simulink library "halin"  (R2021b)
settings: Solver=VariableStepAuto  StartTime=0.0  StopTime=10.0  RelTol=1e-3
undefined symbols (not defined in the file): KHAL_CAN1ABM1E2E_flg, KHAL_CAN1ESC1E2E_flg, KHAL_CAN1ESC5E2E_flg, KHAL_CAN1ESC7E2E_flg, KHAL_CAN1FCM2E2E_flg, KHAL_CAN1FCM3E2E_flg, KHAL_CAN1FCM4E2E_flg, KHAL_CAN3BMS1E2E_flg, KHAL_CAN3BMS6E2E_flg, KHAL_CAN3CCU1E2E_flg, KHAL_CAN3CCU2E2E_flg, KHAL_CAN3MCUF1E2E_flg, KHAL_CAN3MCUR1E2E_flg, KHAL_CAN3Shifter1E2E_flg, TRUE
libraries: simulink x420, FVT_lib x149, hcu_lib x49
(part 7 of 14)

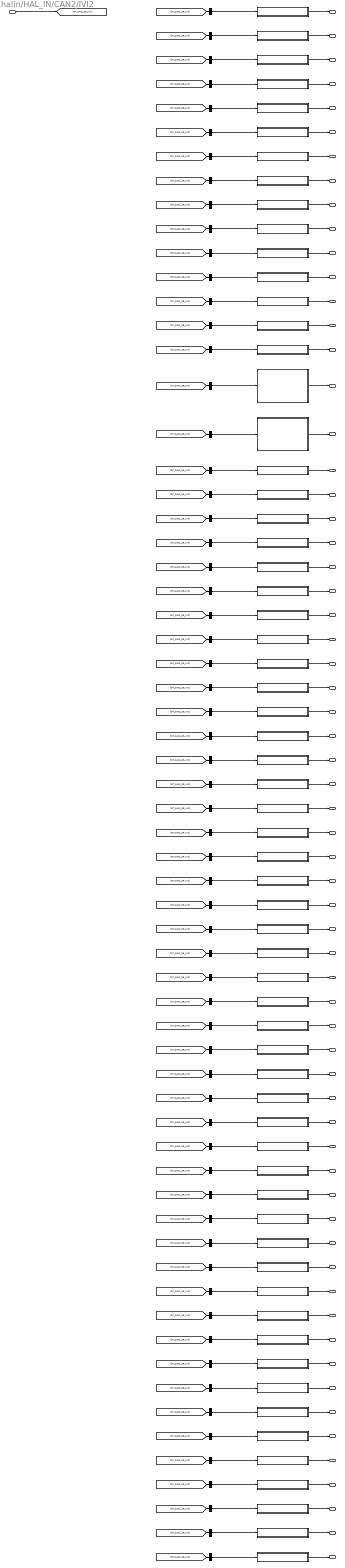
== system halin/HAL_IN/CAN2/IVI2 ==
  DT_CAN2_SG_IVI2 : Inport
  AVMErrSTA : Subsystem
  AVMOFFRecButt : Subsystem
  AVMParkingmode : Subsystem
  AVMparkingcancel : Subsystem
  AVMparkingexcute : Subsystem
  ApproachUnlockSW : Subsystem
  CAASSw : Subsystem
  CDLLockButt : Subsystem
  CDLUnlockButt : Subsystem
  DSEATantiset : Subsystem
  DSEATentryfunset : Subsystem
  DSEATventreq : Subsystem
  ESCSWCmd : Subsystem
  FSOffSw : Subsystem
  FollowMeSW : Subsystem
  GPSLAT : Subsystem
  GPSLONG : Subsystem
  HeadLampSW : Subsystem
  HoodLatchSW : Subsystem
  IVICreepSWReq : Subsystem
  IVIISAOffsetSpd : Subsystem
  IVINightModeSta : Subsystem
  IVIPTGModeSW : Subsystem
  IVIPTGOpenHeight : Subsystem
  IVIPTGStaSW : Subsystem
  IVIPTGUSStaSW : Subsystem
  IVIPWModeReq : Subsystem
  IVIPwrLockSW : Subsystem
  IVIPwroffreq : Subsystem
  IVIRRDefReq : Subsystem
  IVIReqV2L : Subsystem
  IVIScreen : Subsystem
  IVIStatus : Subsystem
  IVITriggerreq : Subsystem
  IVIWIMAINSW : Subsystem
  LDrvControlCommand : Subsystem
  LPasControlCommand : Subsystem
  LRLDControlCommand : Subsystem
  LRRDControlCommand : Subsystem
  MFRDNBrightReq : Subsystem
  OFFACMODE : Subsystem
  PSEATventreq : Subsystem
  PerdV2L : Subsystem
  RFogLampSW : Subsystem
  RollModeSWCmd : Subsystem
  RoomLampMode : Subsystem
  SOCV2LLimit : Subsystem
  SchedChgbutt : Subsystem
  SchedChgwake : Subsystem
  SenstivityPosition : Subsystem
  SetUnlockSingle : Subsystem
  TCSSWCmd : Subsystem
  TPMSCaliButt : Subsystem
  TPMSResButt : Subsystem
  TurnSwTimeSet : Subsystem
  WalkawayLockSW : Subsystem
  bus_selector : BusSelector  OutputSignals=CAN2_AVM_Err_STA
  bus_selector1 : BusSelector  OutputSignals=CAN2_AVM_OFF_Rec_Butt
  bus_selector10 : BusSelector  OutputSignals=CAN2_DSEAT_entryfun_set
  bus_selector11 : BusSelector  OutputSignals=CAN2_DSEAT_vent_req
  bus_selector12 : BusSelector  OutputSignals=CAN2_ESC_SW_Cmd
  bus_selector13 : BusSelector  OutputSignals=CAN2_FS_Off_Sw
  bus_selector14 : BusSelector  OutputSignals=CAN2_FollowMeSW
  bus_selector15 : BusSelector  OutputSignals=CAN2_GPS_LAT
  bus_selector16 : BusSelector  OutputSignals=CAN2_GPS_LONG
  bus_selector17 : BusSelector  OutputSignals=CAN2_HeadLampSW
  bus_selector18 : BusSelector  OutputSignals=CAN2_Hood_Latch_SW
  bus_selector19 : BusSelector  OutputSignals=CAN2_IVI_CreepSW_Req
  bus_selector2 : BusSelector  OutputSignals=CAN2_AVM_Parking_mode
  bus_selector20 : BusSelector  OutputSignals=CAN2_IVI_ISA_OffsetSpd
  bus_selector21 : BusSelector  OutputSignals=CAN2_IVI_Night_Mode_Sta
  bus_selector22 : BusSelector  OutputSignals=CAN2_IVI_PTG_Mode_SW
  bus_selector23 : BusSelector  OutputSignals=CAN2_IVI_PTG_Open_Height
  bus_selector24 : BusSelector  OutputSignals=CAN2_IVI_PTG_Sta_SW
  bus_selector25 : BusSelector  OutputSignals=CAN2_IVI_PTG_USSta_SW
  bus_selector26 : BusSelector  OutputSignals=CAN2_IVI_PW_Mode_Req
  bus_selector27 : BusSelector  OutputSignals=CAN2_IVI_PwrLockSW
  bus_selector28 : BusSelector  OutputSignals=CAN2_IVI_Pwroff_req
  bus_selector29 : BusSelector  OutputSignals=CAN2_IVI_RR_Def_Req
  bus_selector3 : BusSelector  OutputSignals=CAN2_AVM_parking_cancel
  bus_selector30 : BusSelector  OutputSignals=CAN2_IVI_Req_V2L
  bus_selector31 : BusSelector  OutputSignals=CAN2_IVI_Screen
  bus_selector32 : BusSelector  OutputSignals=CAN2_IVI_Status
  bus_selector33 : BusSelector  OutputSignals=CAN2_IVI_Trigger_req
  bus_selector34 : BusSelector  OutputSignals=CAN2_IVI_WI_MAIN_SW
  bus_selector35 : BusSelector  OutputSignals=CAN2_L_Drv_ControlCommand
  bus_selector36 : BusSelector  OutputSignals=CAN2_L_Pas_ControlCommand
  bus_selector37 : BusSelector  OutputSignals=CAN2_L_RLD_ControlCommand
  bus_selector38 : BusSelector  OutputSignals=CAN2_L_RRD_ControlCommand
  bus_selector39 : BusSelector  OutputSignals=CAN2_MFRD_N_Bright_Req
  bus_selector4 : BusSelector  OutputSignals=CAN2_AVM_parking_excute
  bus_selector40 : BusSelector  OutputSignals=CAN2_OFF_AC_MODE
  bus_selector41 : BusSelector  OutputSignals=CAN2_PSEAT_vent_req
  bus_selector42 : BusSelector  OutputSignals=CAN2_Perd_V2L
  bus_selector43 : BusSelector  OutputSignals=CAN2_RFogLampSW
  bus_selector44 : BusSelector  OutputSignals=CAN2_Roll_Mode_SW_Cmd
  bus_selector45 : BusSelector  OutputSignals=CAN2_RoomLampMode
  bus_selector46 : BusSelector  OutputSignals=CAN2_SOC_V2LLimit
  bus_selector47 : BusSelector  OutputSignals=CAN2_Sched_Chg_butt
  bus_selector48 : BusSelector  OutputSignals=CAN2_Sched_Chg_wake
  bus_selector49 : BusSelector  OutputSignals=CAN2_SenstivityPosition
  bus_selector5 : BusSelector  OutputSignals=CAN2_Approach_Unlock_SW
  bus_selector50 : BusSelector  OutputSignals=CAN2_SetUnlockSingle
  bus_selector51 : BusSelector  OutputSignals=CAN2_TCS_SW_Cmd
  bus_selector52 : BusSelector  OutputSignals=CAN2_TPMS_Cali_Butt
  bus_selector53 : BusSelector  OutputSignals=CAN2_TPMS_Res_Butt
  bus_selector54 : BusSelector  OutputSignals=CAN2_TurnSwTimeSet
  bus_selector55 : BusSelector  OutputSignals=CAN2_Walkaway_Lock_SW
  bus_selector56 : BusSelector  OutputSignals=CAN2_sigAirIntenZon1Req
  bus_selector57 : BusSelector  OutputSignals=CAN2_sigDfrstReq
  bus_selector58 : BusSelector  OutputSignals=CAN2_sigFaceReq
  bus_selector59 : BusSelector  OutputSignals=CAN2_sigFootReq
  bus_selector6 : BusSelector  OutputSignals=CAN2_CAAS_Sw
  bus_selector60 : BusSelector  OutputSignals=CAN2_sigRecircReq
  bus_selector61 : BusSelector  OutputSignals=CAN2_sigSetTempZon1Req
  bus_selector62 : BusSelector  OutputSignals=CAN2_sigSetTempZon2Req
  bus_selector7 : BusSelector  OutputSignals=CAN2_CDL_Lock_Butt
  bus_selector8 : BusSelector  OutputSignals=CAN2_CDL_Unlock_Butt
  bus_selector9 : BusSelector  OutputSignals=CAN2_DSEAT_anti_set
  sigAirIntenZon1Req : Subsystem
  sigDfrstReq : Subsystem
  sigFaceReq : Subsystem
  sigFootReq : Subsystem
  sigRecircReq : Subsystem
  sigSetTempZon1Req : Subsystem
  sigSetTempZon2Req : Subsystem
  VHAL_AVMErrSTA_flg : Outport
  VHAL_AVMOFFRecButt_flg : Outport  Port=2
  VHAL_AVMParkingmode_enum : Outport  Port=3
  VHAL_AVMparkingcancel_enum : Outport  Port=4
  VHAL_AVMparkingexcute_enum : Outport  Port=5
  VHAL_ApproachUnlockSW_flg : Outport  Port=6
  VHAL_CAASSw_enum : Outport  Port=7
  VHAL_CDLLockButt_flg : Outport  Port=8
  VHAL_CDLUnlockButt_flg : Outport  Port=9
  VHAL_DSEATantiset_flg : Outport  Port=10
  VHAL_DSEATentryfunset_flg : Outport  Port=11
  VHAL_DSEATventreq_enum : Outport  Port=12
  VHAL_ESCSWCmd_enum : Outport  Port=13
  VHAL_FSOffSw_enum : Outport  Port=14
  VHAL_FollowMeSW_flg : Outport  Port=15
  VHAL_GPSLAT_s : Outport  Port=16
  VHAL_GPSLONG_enum : Outport  Port=17
  VHAL_HeadLampSW_enum : Outport  Port=18
  VHAL_HoodLatchSW_enum : Outport  Port=19
  VHAL_IVICreepSWReq_flg : Outport  Port=20
  VHAL_IVIISAOffsetSpd_enum : Outport  Port=21
  VHAL_IVINightModeSta_flg : Outport  Port=22
  VHAL_IVIPTGModeSW_enum : Outport  Port=23
  VHAL_IVIPTGOpenHeight_enum : Outport  Port=24
  VHAL_IVIPTGStaSW_enum : Outport  Port=25
  VHAL_IVIPTGUSStaSW_flg : Outport  Port=26
  VHAL_IVIPWModeReq_enum : Outport  Port=27
  VHAL_IVIPwrLockSW_enum : Outport  Port=28
  VHAL_IVIPwroffreq_flg : Outport  Port=29
  VHAL_IVIRRDefReq_flg : Outport  Port=30
  VHAL_IVIReqV2L_flg : Outport  Port=31
  VHAL_IVIScreen_enum : Outport  Port=32
  VHAL_IVIStatus_flg : Outport  Port=33
  VHAL_IVITriggerreq_flg : Outport  Port=34
  VHAL_IVIWIMAINSW_flg : Outport  Port=35
  VHAL_LDrvControlCommand_pct : Outport  Port=36
  VHAL_LPasControlCommand_pct : Outport  Port=37
  VHAL_LRLDControlCommand_pct : Outport  Port=38
  VHAL_LRRDControlCommand_pct : Outport  Port=39
  VHAL_MFRDNBrightReq_pct : Outport  Port=40
  VHAL_OFFACMODE_enum : Outport  Port=41
  VHAL_PSEATventreq_enum : Outport  Port=42
  VHAL_PerdV2L_enum : Outport  Port=43
  VHAL_RFogLampSW_flg : Outport  Port=44
  VHAL_RollModeSWCmd_enum : Outport  Port=45
  VHAL_RoomLampMode_flg : Outport  Port=46
  VHAL_SOCV2LLimit_pct : Outport  Port=47
  VHAL_SchedChgbutt_flg : Outport  Port=48
  VHAL_SchedChgwake_flg : Outport  Port=49
  VHAL_SenstivityPosition_enum : Outport  Port=50
  VHAL_SetUnlockSingle_flg : Outport  Port=51
  VHAL_TCSSWCmd_enum : Outport  Port=52
  VHAL_TPMSCaliButt_flg : Outport  Port=53
  VHAL_TPMSResButt_flg : Outport  Port=54
  VHAL_TurnSwTimeSet_enum : Outport  Port=55
  VHAL_WalkawayLockSW_flg : Outport  Port=56
  VHAL_sigAirIntenZon1Req_enum : Outport  Port=57
  VHAL_sigDfrstReq_flg : Outport  Port=58
  VHAL_sigFaceReq_flg : Outport  Port=59
  VHAL_sigFootReq_flg : Outport  Port=60
  VHAL_sigRecircReq_flg : Outport  Port=61
  VHAL_sigSetTempZon1Req_C : Outport  Port=62
  VHAL_sigSetTempZon2Req_C : Outport  Port=63
  wires:
  DT_CAN2_SG_IVI2/1 -> [DT_CAN2_SG_IVI2]
  [DT_CAN2_SG_IVI2] -> bus_selector/1
  bus_selector/1 -> AVMErrSTA/1(AVM_Err_STA)  "<CAN2_AVM_Err_STA>"
  AVMErrSTA/1(VHAL_AVMErrSTA_flg) -> VHAL_AVMErrSTA_flg/1
  [DT_CAN2_SG_IVI2] -> bus_selector1/1
  bus_selector1/1 -> AVMOFFRecButt/1(AVM_OFF_Rec_Butt)  "<CAN2_AVM_OFF_Rec_Butt>"
  AVMOFFRecButt/1(VHAL_AVMOFFRecButt_flg) -> VHAL_AVMOFFRecButt_flg/1
  [DT_CAN2_SG_IVI2] -> bus_selector2/1
  bus_selector2/1 -> AVMParkingmode/1(AVM_Parking_mode)  "<CAN2_AVM_Parking_mode>"
  AVMParkingmode/1(VHAL_AVMParkingmode_enum) -> VHAL_AVMParkingmode_enum/1
  [DT_CAN2_SG_IVI2] -> bus_selector3/1
  bus_selector3/1 -> AVMparkingcancel/1(AVM_parking_cancel)  "<CAN2_AVM_parking_cancel>"
  AVMparkingcancel/1(VHAL_AVMparkingcancel_enum) -> VHAL_AVMparkingcancel_enum/1
  [DT_CAN2_SG_IVI2] -> bus_selector4/1
  bus_selector4/1 -> AVMparkingexcute/1(AVM_parking_excute)  "<CAN2_AVM_parking_excute>"
  AVMparkingexcute/1(VHAL_AVMparkingexcute_enum) -> VHAL_AVMparkingexcute_enum/1
  [DT_CAN2_SG_IVI2] -> bus_selector5/1
  bus_selector5/1 -> ApproachUnlockSW/1(Approach_Unlock_SW)  "<CAN2_Approach_Unlock_SW>"
  ApproachUnlockSW/1(VHAL_ApproachUnlockSW_flg) -> VHAL_ApproachUnlockSW_flg/1
  [DT_CAN2_SG_IVI2] -> bus_selector6/1
  bus_selector6/1 -> CAASSw/1(CAAS_Sw)  "<CAN2_CAAS_Sw>"
  CAASSw/1(VHAL_CAASSw_enum) -> VHAL_CAASSw_enum/1
  [DT_CAN2_SG_IVI2] -> bus_selector7/1
  bus_selector7/1 -> CDLLockButt/1(CDL_Lock_Butt)  "<CAN2_CDL_Lock_Butt>"
  CDLLockButt/1(VHAL_CDLLockButt_flg) -> VHAL_CDLLockButt_flg/1
  [DT_CAN2_SG_IVI2] -> bus_selector8/1
  bus_selector8/1 -> CDLUnlockButt/1(CDL_Unlock_Butt)  "<CAN2_CDL_Unlock_Butt>"
  CDLUnlockButt/1(VHAL_CDLUnlockButt_flg) -> VHAL_CDLUnlockButt_flg/1
  [DT_CAN2_SG_IVI2] -> bus_selector9/1
  bus_selector9/1 -> DSEATantiset/1(DSEAT_anti_set)  "<CAN2_DSEAT_anti_set>"
  DSEATantiset/1(VHAL_DSEATantiset_flg) -> VHAL_DSEATantiset_flg/1
  [DT_CAN2_SG_IVI2] -> bus_selector10/1
  bus_selector10/1 -> DSEATentryfunset/1(DSEAT_entryfun_set)  "<CAN2_DSEAT_entryfun_set>"
  DSEATentryfunset/1(VHAL_DSEATentryfunset_flg) -> VHAL_DSEATentryfunset_flg/1
  [DT_CAN2_SG_IVI2] -> bus_selector11/1
  bus_selector11/1 -> DSEATventreq/1(DSEAT_vent_req)  "<CAN2_DSEAT_vent_req>"
  DSEATventreq/1(VHAL_DSEATventreq_enum) -> VHAL_DSEATventreq_enum/1
  [DT_CAN2_SG_IVI2] -> bus_selector12/1
  bus_selector12/1 -> ESCSWCmd/1(ESC_SW_Cmd)  "<CAN2_ESC_SW_Cmd>"
  ESCSWCmd/1(VHAL_ESCSWCmd_enum) -> VHAL_ESCSWCmd_enum/1
  [DT_CAN2_SG_IVI2] -> bus_selector13/1
  bus_selector13/1 -> FSOffSw/1(FS_Off_Sw)  "<CAN2_FS_Off_Sw>"
  FSOffSw/1(VHAL_FSOffSw_enum) -> VHAL_FSOffSw_enum/1
  [DT_CAN2_SG_IVI2] -> bus_selector14/1
  bus_selector14/1 -> FollowMeSW/1(FollowMeSW)  "<CAN2_FollowMeSW>"
  FollowMeSW/1(VHAL_FollowMeSW_flg) -> VHAL_FollowMeSW_flg/1
  [DT_CAN2_SG_IVI2] -> bus_selector15/1
  bus_selector15/1 -> GPSLAT/1(GPS_LAT)  "<CAN2_GPS_LAT>"
  GPSLAT/1(VHAL_GPSLAT_s) -> VHAL_GPSLAT_s/1
  [DT_CAN2_SG_IVI2] -> bus_selector16/1
  bus_selector16/1 -> GPSLONG/1(GPS_LONG)  "<CAN2_GPS_LONG>"
  GPSLONG/1(VHAL_GPSLONG_enum) -> VHAL_GPSLONG_enum/1
  [DT_CAN2_SG_IVI2] -> bus_selector17/1
  bus_selector17/1 -> HeadLampSW/1(HeadLampSW)  "<CAN2_HeadLampSW>"
  HeadLampSW/1(VHAL_HeadLampSW_enum) -> VHAL_HeadLampSW_enum/1
  [DT_CAN2_SG_IVI2] -> bus_selector18/1
  bus_selector18/1 -> HoodLatchSW/1(Hood_Latch_SW)  "<CAN2_Hood_Latch_SW>"
  HoodLatchSW/1(VHAL_HoodLatchSW_enum) -> VHAL_HoodLatchSW_enum/1
  [DT_CAN2_SG_IVI2] -> bus_selector19/1
  bus_selector19/1 -> IVICreepSWReq/1(IVI_CreepSW_Req)  "<CAN2_IVI_CreepSW_Req>"
  IVICreepSWReq/1(VHAL_IVICreepSWReq_flg) -> VHAL_IVICreepSWReq_flg/1
  [DT_CAN2_SG_IVI2] -> bus_selector20/1
  bus_selector20/1 -> IVIISAOffsetSpd/1(IVI_ISA_OffsetSpd)  "<CAN2_IVI_ISA_OffsetSpd>"
  IVIISAOffsetSpd/1(VHAL_IVIISAOffsetSpd_enum) -> VHAL_IVIISAOffsetSpd_enum/1
  [DT_CAN2_SG_IVI2] -> bus_selector21/1
  bus_selector21/1 -> IVINightModeSta/1(IVI_Night_Mode_Sta)  "<CAN2_IVI_Night_Mode_Sta>"
  IVINightModeSta/1(VHAL_IVINightModeSta_flg) -> VHAL_IVINightModeSta_flg/1
  [DT_CAN2_SG_IVI2] -> bus_selector22/1
  bus_selector22/1 -> IVIPTGModeSW/1(IVI_PTG_Mode_SW)  "<CAN2_IVI_PTG_Mode_SW>"
  IVIPTGModeSW/1(VHAL_IVIPTGModeSW_enum) -> VHAL_IVIPTGModeSW_enum/1
  [DT_CAN2_SG_IVI2] -> bus_selector23/1
  bus_selector23/1 -> IVIPTGOpenHeight/1(IVI_PTG_Open_Height)  "<CAN2_IVI_PTG_Open_Height>"
  IVIPTGOpenHeight/1(VHAL_IVIPTGOpenHeight_enum) -> VHAL_IVIPTGOpenHeight_enum/1
  [DT_CAN2_SG_IVI2] -> bus_selector24/1
  bus_selector24/1 -> IVIPTGStaSW/1(IVI_PTG_Sta_SW)  "<CAN2_IVI_PTG_Sta_SW>"
  IVIPTGStaSW/1(VHAL_IVIPTGStaSW_enum) -> VHAL_IVIPTGStaSW_enum/1
  [DT_CAN2_SG_IVI2] -> bus_selector25/1
  bus_selector25/1 -> IVIPTGUSStaSW/1(IVI_PTG_USSta_SW)  "<CAN2_IVI_PTG_USSta_SW>"
  IVIPTGUSStaSW/1(VHAL_IVIPTGUSStaSW_flg) -> VHAL_IVIPTGUSStaSW_flg/1
  [DT_CAN2_SG_IVI2] -> bus_selector26/1
  bus_selector26/1 -> IVIPWModeReq/1(IVI_PW_Mode_Req)  "<CAN2_IVI_PW_Mode_Req>"
  IVIPWModeReq/1(VHAL_IVIPWModeReq_enum) -> VHAL_IVIPWModeReq_enum/1
  [DT_CAN2_SG_IVI2] -> bus_selector27/1
  bus_selector27/1 -> IVIPwrLockSW/1(IVI_PwrLockSW)  "<CAN2_IVI_PwrLockSW>"
  IVIPwrLockSW/1(VHAL_IVIPwrLockSW_enum) -> VHAL_IVIPwrLockSW_enum/1
  [DT_CAN2_SG_IVI2] -> bus_selector28/1
  bus_selector28/1 -> IVIPwroffreq/1(IVI_Pwroff_req)  "<CAN2_IVI_Pwroff_req>"
  IVIPwroffreq/1(VHAL_IVIPwroffreq_flg) -> VHAL_IVIPwroffreq_flg/1
  [DT_CAN2_SG_IVI2] -> bus_selector29/1
  bus_selector29/1 -> IVIRRDefReq/1(IVI_RR_Def_Req)  "<CAN2_IVI_RR_Def_Req>"
  IVIRRDefReq/1(VHAL_IVIRRDefReq_flg) -> VHAL_IVIRRDefReq_flg/1
  [DT_CAN2_SG_IVI2] -> bus_selector30/1
  bus_selector30/1 -> IVIReqV2L/1(IVI_Req_V2L)  "<CAN2_IVI_Req_V2L>"
  IVIReqV2L/1(VHAL_IVIReqV2L_flg) -> VHAL_IVIReqV2L_flg/1
  [DT_CAN2_SG_IVI2] -> bus_selector31/1
  bus_selector31/1 -> IVIScreen/1(IVI_Screen)  "<CAN2_IVI_Screen>"
  IVIScreen/1(VHAL_IVIScreen_enum) -> VHAL_IVIScreen_enum/1
  [DT_CAN2_SG_IVI2] -> bus_selector32/1
  bus_selector32/1 -> IVIStatus/1(IVI_Status)  "<CAN2_IVI_Status>"
  IVIStatus/1(VHAL_IVIStatus_flg) -> VHAL_IVIStatus_flg/1
  [DT_CAN2_SG_IVI2] -> bus_selector33/1
  bus_selector33/1 -> IVITriggerreq/1(IVI_Trigger_req)  "<CAN2_IVI_Trigger_req>"
  IVITriggerreq/1(VHAL_IVITriggerreq_flg) -> VHAL_IVITriggerreq_flg/1
  [DT_CAN2_SG_IVI2] -> bus_selector34/1
  bus_selector34/1 -> IVIWIMAINSW/1(IVI_WI_MAIN_SW)  "<CAN2_IVI_WI_MAIN_SW>"
  IVIWIMAINSW/1(VHAL_IVIWIMAINSW_flg) -> VHAL_IVIWIMAINSW_flg/1
  [DT_CAN2_SG_IVI2] -> bus_selector35/1
  bus_selector35/1 -> LDrvControlCommand/1(L_Drv_ControlCommand)  "<CAN2_L_Drv_ControlCommand>"
  LDrvControlCommand/1(VHAL_LDrvControlCommand_pct) -> VHAL_LDrvControlCommand_pct/1
  [DT_CAN2_SG_IVI2] -> bus_selector36/1
  bus_selector36/1 -> LPasControlCommand/1(L_Pas_ControlCommand)  "<CAN2_L_Pas_ControlCommand>"
  LPasControlCommand/1(VHAL_LPasControlCommand_pct) -> VHAL_LPasControlCommand_pct/1
  [DT_CAN2_SG_IVI2] -> bus_selector37/1
  bus_selector37/1 -> LRLDControlCommand/1(L_RLD_ControlCommand)  "<CAN2_L_RLD_ControlCommand>"
  LRLDControlCommand/1(VHAL_LRLDControlCommand_pct) -> VHAL_LRLDControlCommand_pct/1
  [DT_CAN2_SG_IVI2] -> bus_selector38/1
  bus_selector38/1 -> LRRDControlCommand/1(L_RRD_ControlCommand)  "<CAN2_L_RRD_ControlCommand>"
  LRRDControlCommand/1(VHAL_LRRDControlCommand_pct) -> VHAL_LRRDControlCommand_pct/1
  [DT_CAN2_SG_IVI2] -> bus_selector39/1
  bus_selector39/1 -> MFRDNBrightReq/1(MFRD_N_Bright_Req)  "<CAN2_MFRD_N_Bright_Req>"
  MFRDNBrightReq/1(VHAL_MFRDNBrightReq_pct) -> VHAL_MFRDNBrightReq_pct/1
  [DT_CAN2_SG_IVI2] -> bus_selector40/1
  bus_selector40/1 -> OFFACMODE/1(OFF_AC_MODE)  "<CAN2_OFF_AC_MODE>"
  OFFACMODE/1(VHAL_OFFACMODE_enum) -> VHAL_OFFACMODE_enum/1
  [DT_CAN2_SG_IVI2] -> bus_selector41/1
  bus_selector41/1 -> PSEATventreq/1(PSEAT_vent_req)  "<CAN2_PSEAT_vent_req>"
  PSEATventreq/1(VHAL_PSEATventreq_enum) -> VHAL_PSEATventreq_enum/1
  [DT_CAN2_SG_IVI2] -> bus_selector42/1
  bus_selector42/1 -> PerdV2L/1(Perd_V2L)  "<CAN2_Perd_V2L>"
  PerdV2L/1(VHAL_PerdV2L_enum) -> VHAL_PerdV2L_enum/1
  [DT_CAN2_SG_IVI2] -> bus_selector43/1
  bus_selector43/1 -> RFogLampSW/1(RFogLampSW)  "<CAN2_RFogLampSW>"
  RFogLampSW/1(VHAL_RFogLampSW_flg) -> VHAL_RFogLampSW_flg/1
  [DT_CAN2_SG_IVI2] -> bus_selector44/1
  bus_selector44/1 -> RollModeSWCmd/1(Roll_Mode_SW_Cmd)  "<CAN2_Roll_Mode_SW_Cmd>"
  RollModeSWCmd/1(VHAL_RollModeSWCmd_enum) -> VHAL_RollModeSWCmd_enum/1
  [DT_CAN2_SG_IVI2] -> bus_selector45/1
  bus_selector45/1 -> RoomLampMode/1(RoomLampMode)  "<CAN2_RoomLampMode>"
  RoomLampMode/1(VHAL_RoomLampMode_flg) -> VHAL_RoomLampMode_flg/1
  [DT_CAN2_SG_IVI2] -> bus_selector46/1
  bus_selector46/1 -> SOCV2LLimit/1(SOC_V2LLimit)  "<CAN2_SOC_V2LLimit>"
  SOCV2LLimit/1(VHAL_SOCV2LLimit_pct) -> VHAL_SOCV2LLimit_pct/1
  [DT_CAN2_SG_IVI2] -> bus_selector47/1
  bus_selector47/1 -> SchedChgbutt/1(Sched_Chg_butt)  "<CAN2_Sched_Chg_butt>"
  SchedChgbutt/1(VHAL_SchedChgbutt_flg) -> VHAL_SchedChgbutt_flg/1
  [DT_CAN2_SG_IVI2] -> bus_selector48/1
  bus_selector48/1 -> SchedChgwake/1(Sched_Chg_wake)  "<CAN2_Sched_Chg_wake>"
  SchedChgwake/1(VHAL_SchedChgwake_flg) -> VHAL_SchedChgwake_flg/1
  [DT_CAN2_SG_IVI2] -> bus_selector49/1
  bus_selector49/1 -> SenstivityPosition/1(SenstivityPosition)  "<CAN2_SenstivityPosition>"
  SenstivityPosition/1(VHAL_SenstivityPosition_enum) -> VHAL_SenstivityPosition_enum/1
  [DT_CAN2_SG_IVI2] -> bus_selector50/1
  bus_selector50/1 -> SetUnlockSingle/1(SetUnlockSingle)  "<CAN2_SetUnlockSingle>"
  SetUnlockSingle/1(VHAL_SetUnlockSingle_flg) -> VHAL_SetUnlockSingle_flg/1
  [DT_CAN2_SG_IVI2] -> bus_selector51/1
  bus_selector51/1 -> TCSSWCmd/1(TCS_SW_Cmd)  "<CAN2_TCS_SW_Cmd>"
  TCSSWCmd/1(VHAL_TCSSWCmd_enum) -> VHAL_TCSSWCmd_enum/1
  [DT_CAN2_SG_IVI2] -> bus_selector52/1
  bus_selector52/1 -> TPMSCaliButt/1(TPMS_Cali_Butt)  "<CAN2_TPMS_Cali_Butt>"
  TPMSCaliButt/1(VHAL_TPMSCaliButt_flg) -> VHAL_TPMSCaliButt_flg/1
  [DT_CAN2_SG_IVI2] -> bus_selector53/1
  bus_selector53/1 -> TPMSResButt/1(TPMS_Res_Butt)  "<CAN2_TPMS_Res_Butt>"
  TPMSResButt/1(VHAL_TPMSResButt_flg) -> VHAL_TPMSResButt_flg/1
  [DT_CAN2_SG_IVI2] -> bus_selector54/1
  bus_selector54/1 -> TurnSwTimeSet/1(TurnSwTimeSet)  "<CAN2_TurnSwTimeSet>"
  TurnSwTimeSet/1(VHAL_TurnSwTimeSet_enum) -> VHAL_TurnSwTimeSet_enum/1
  [DT_CAN2_SG_IVI2] -> bus_selector55/1
  bus_selector55/1 -> WalkawayLockSW/1(Walkaway_Lock_SW)  "<CAN2_Walkaway_Lock_SW>"
  WalkawayLockSW/1(VHAL_WalkawayLockSW_flg) -> VHAL_WalkawayLockSW_flg/1
  [DT_CAN2_SG_IVI2] -> bus_selector56/1
  bus_selector56/1 -> sigAirIntenZon1Req/1(sigAirIntenZon1Req)  "<CAN2_sigAirIntenZon1Req>"
  sigAirIntenZon1Req/1(VHAL_sigAirIntenZon1Req_enum) -> VHAL_sigAirIntenZon1Req_enum/1
  [DT_CAN2_SG_IVI2] -> bus_selector57/1
  bus_selector57/1 -> sigDfrstReq/1(sigDfrstReq)  "<CAN2_sigDfrstReq>"
  sigDfrstReq/1(VHAL_sigDfrstReq_flg) -> VHAL_sigDfrstReq_flg/1
  [DT_CAN2_SG_IVI2] -> bus_selector58/1
  bus_selector58/1 -> sigFaceReq/1(sigFaceReq)  "<CAN2_sigFaceReq>"
  sigFaceReq/1(VHAL_sigFaceReq_flg) -> VHAL_sigFaceReq_flg/1
  [DT_CAN2_SG_IVI2] -> bus_selector59/1
  bus_selector59/1 -> sigFootReq/1(sigFootReq)  "<CAN2_sigFootReq>"
  sigFootReq/1(VHAL_sigFootReq_flg) -> VHAL_sigFootReq_flg/1
  [DT_CAN2_SG_IVI2] -> bus_selector60/1
  bus_selector60/1 -> sigRecircReq/1(sigRecircReq)  "<CAN2_sigRecircReq>"
  sigRecircReq/1(VHAL_sigRecircReq_flg) -> VHAL_sigRecircReq_flg/1
  [DT_CAN2_SG_IVI2] -> bus_selector61/1
  bus_selector61/1 -> sigSetTempZon1Req/1(sigSetTempZon1Req)  "<CAN2_sigSetTempZon1Req>"
  sigSetTempZon1Req/1(VHAL_sigSetTempZon1Req_C) -> VHAL_sigSetTempZon1Req_C/1
  [DT_CAN2_SG_IVI2] -> bus_selector62/1
  bus_selector62/1 -> sigSetTempZon2Req/1(sigSetTempZon2Req)  "<CAN2_sigSetTempZon2Req>"
  sigSetTempZon2Req/1(VHAL_sigSetTempZon2Req_C) -> VHAL_sigSetTempZon2Req_C/1

== system halin/HAL_IN/CAN2/IVI6 ==
  DT_CAN2_SG_IVI6 : Inport
  IVILocatedSTA : Subsystem
  IVITimeCheck : Subsystem
  IVITimeDay : Subsystem
  IVITimeHour : Subsystem
  IVITimeMinute : Subsystem
  IVITimeMonth : Subsystem
  IVITimeSecond : Subsystem
  IVITimeYear : Subsystem
  bus_selector : BusSelector  OutputSignals=CAN2_IVI_Located_STA
  bus_selector1 : BusSelector  OutputSignals=CAN2_IVI_Time_Check
  bus_selector2 : BusSelector  OutputSignals=CAN2_IVI_Time_Day
  bus_selector3 : BusSelector  OutputSignals=CAN2_IVI_Time_Hour
  bus_selector4 : BusSelector  OutputSignals=CAN2_IVI_Time_Minute
  bus_selector5 : BusSelector  OutputSignals=CAN2_IVI_Time_Month
  bus_selector6 : BusSelector  OutputSignals=CAN2_IVI_Time_Second
  bus_selector7 : BusSelector  OutputSignals=CAN2_IVI_Time_Year
  VHAL_IVILocatedSTA_enum : Outport
  VHAL_IVITimeCheck_enum : Outport  Port=2
  VHAL_IVITimeDay_DAY : Outport  Port=3
  VHAL_IVITimeHour_hr : Outport  Port=4
  VHAL_IVITimeMinute_min : Outport  Port=5
  VHAL_IVITimeMonth_MONTH : Outport  Port=6
  VHAL_IVITimeSecond_s : Outport  Port=7
  VHAL_IVITimeYear_YEAR : Outport  Port=8
  wires:
  DT_CAN2_SG_IVI6/1 -> [DT_CAN2_SG_IVI6]
  [DT_CAN2_SG_IVI6] -> bus_selector/1
  bus_selector/1 -> IVILocatedSTA/1(IVI_Located_STA)  "<CAN2_IVI_Located_STA>"
  IVILocatedSTA/1(VHAL_IVILocatedSTA_enum) -> VHAL_IVILocatedSTA_enum/1
  [DT_CAN2_SG_IVI6] -> bus_selector1/1
  bus_selector1/1 -> IVITimeCheck/1(IVI_Time_Check)  "<CAN2_IVI_Time_Check>"
  IVITimeCheck/1(VHAL_IVITimeCheck_enum) -> VHAL_IVITimeCheck_enum/1
  [DT_CAN2_SG_IVI6] -> bus_selector2/1
  bus_selector2/1 -> IVITimeDay/1(IVI_Time_Day)  "<CAN2_IVI_Time_Day>"
  IVITimeDay/1(VHAL_IVITimeDay_DAY) -> VHAL_IVITimeDay_DAY/1
  [DT_CAN2_SG_IVI6] -> bus_selector3/1
  bus_selector3/1 -> IVITimeHour/1(IVI_Time_Hour)  "<CAN2_IVI_Time_Hour>"
  IVITimeHour/1(VHAL_IVITimeHour_hr) -> VHAL_IVITimeHour_hr/1
  [DT_CAN2_SG_IVI6] -> bus_selector4/1
  bus_selector4/1 -> IVITimeMinute/1(IVI_Time_Minute)  "<CAN2_IVI_Time_Minute>"
  IVITimeMinute/1(VHAL_IVITimeMinute_min) -> VHAL_IVITimeMinute_min/1
  [DT_CAN2_SG_IVI6] -> bus_selector5/1
  bus_selector5/1 -> IVITimeMonth/1(IVI_Time_Month)  "<CAN2_IVI_Time_Month>"
  IVITimeMonth/1(VHAL_IVITimeMonth_MONTH) -> VHAL_IVITimeMonth_MONTH/1
  [DT_CAN2_SG_IVI6] -> bus_selector6/1
  bus_selector6/1 -> IVITimeSecond/1(IVI_Time_Second)  "<CAN2_IVI_Time_Second>"
  IVITimeSecond/1(VHAL_IVITimeSecond_s) -> VHAL_IVITimeSecond_s/1
  [DT_CAN2_SG_IVI6] -> bus_selector7/1
  bus_selector7/1 -> IVITimeYear/1(IVI_Time_Year)  "<CAN2_IVI_Time_Year>"
  IVITimeYear/1(VHAL_IVITimeYear_YEAR) -> VHAL_IVITimeYear_YEAR/1

== system halin/HAL_IN/CAN2/METER1 ==
  DT_CAN2_SG_METER1 : Inport
  METERKPHCalcu : Subsystem
  bus_selector : BusSelector  OutputSignals=CAN2_METER_KPH_Calcu
  VHAL_METERKPHCalcu_kph : Outport
  wires:
  DT_CAN2_SG_METER1/1 -> [DT_CAN2_SG_METER1]
  [DT_CAN2_SG_METER1] -> bus_selector/1
  bus_selector/1 -> METERKPHCalcu/1(METER_KPH_Calcu)  "<CAN2_METER_KPH_Calcu>"
  METERKPHCalcu/1(VHAL_METERKPHCalcu_kph) -> VHAL_METERKPHCalcu_kph/1

== system halin/HAL_IN/CAN2/VHAL_CANMsgInvalidIVI1_flg ==
  Cast To Boolean13 : DataTypeConversion  OutDataTypeStr=boolean
  Constant : Constant  Value=TRUE
  Latch13 : hcu_lib/Basic_Blocks/Latch
  Switch13 : Switch  Criteria=u2 ~= 0
  Unit Delay : UnitDelay  SampleTime=-1  HasFrameUpgradeWarning=on
  UnitConverter : DataTypeConversion  OutDataTypeStr=boolean
  Out : Outport
  wires:
  Constant/1 -> Switch13/3
  Unit Delay/1 -> Cast To Boolean13/1
  Cast To Boolean13/1 -> Switch13/1, Latch13/1
  Switch13/1 -> UnitConverter/1
  Latch13/1 -> Switch13/2
  UnitConverter/1 -> Unit Delay/1, Out/1  "VHAL_CANMsgInvalidIVI1_flg"

== system halin/HAL_IN/CAN2/VHAL_CANMsgInvalidIVI2_flg ==
  Cast To Boolean13 : DataTypeConversion  OutDataTypeStr=boolean
  Constant : Constant  Value=TRUE
  Latch13 : hcu_lib/Basic_Blocks/Latch
  Switch13 : Switch  Criteria=u2 ~= 0
  Unit Delay : UnitDelay  SampleTime=-1  HasFrameUpgradeWarning=on
  UnitConverter : DataTypeConversion  OutDataTypeStr=boolean
  Out : Outport
  wires:
  Constant/1 -> Switch13/3
  Unit Delay/1 -> Cast To Boolean13/1
  Cast To Boolean13/1 -> Switch13/1, Latch13/1
  Switch13/1 -> UnitConverter/1
  Latch13/1 -> Switch13/2
  UnitConverter/1 -> Unit Delay/1, Out/1  "VHAL_CANMsgInvalidIVI2_flg"

== system halin/HAL_IN/CAN2/VHAL_CANMsgInvalidIVI6_flg ==
  Cast To Boolean13 : DataTypeConversion  OutDataTypeStr=boolean
  Constant : Constant  Value=TRUE
  Latch13 : hcu_lib/Basic_Blocks/Latch
  Switch13 : Switch  Criteria=u2 ~= 0
  Unit Delay : UnitDelay  SampleTime=-1  HasFrameUpgradeWarning=on
  UnitConverter : DataTypeConversion  OutDataTypeStr=boolean
  Out : Outport
  wires:
  Constant/1 -> Switch13/3
  Unit Delay/1 -> Cast To Boolean13/1
  Cast To Boolean13/1 -> Switch13/1, Latch13/1
  Switch13/1 -> UnitConverter/1
  Latch13/1 -> Switch13/2
  UnitConverter/1 -> Unit Delay/1, Out/1  "VHAL_CANMsgInvalidIVI6_flg"

== system halin/HAL_IN/CAN2/VHAL_CANMsgInvalidMETER1_flg ==
  Cast To Boolean13 : DataTypeConversion  OutDataTypeStr=boolean
  Constant : Constant  Value=TRUE
  Latch13 : hcu_lib/Basic_Blocks/Latch
  Switch13 : Switch  Criteria=u2 ~= 0
  Unit Delay : UnitDelay  SampleTime=-1  HasFrameUpgradeWarning=on
  UnitConverter : DataTypeConversion  OutDataTypeStr=boolean
  Out : Outport
  wires:
  Constant/1 -> Switch13/3
  Unit Delay/1 -> Cast To Boolean13/1
  Cast To Boolean13/1 -> Switch13/1, Latch13/1
  Switch13/1 -> UnitConverter/1
  Latch13/1 -> Switch13/2
  UnitConverter/1 -> Unit Delay/1, Out/1  "VHAL_CANMsgInvalidMETER1_flg"

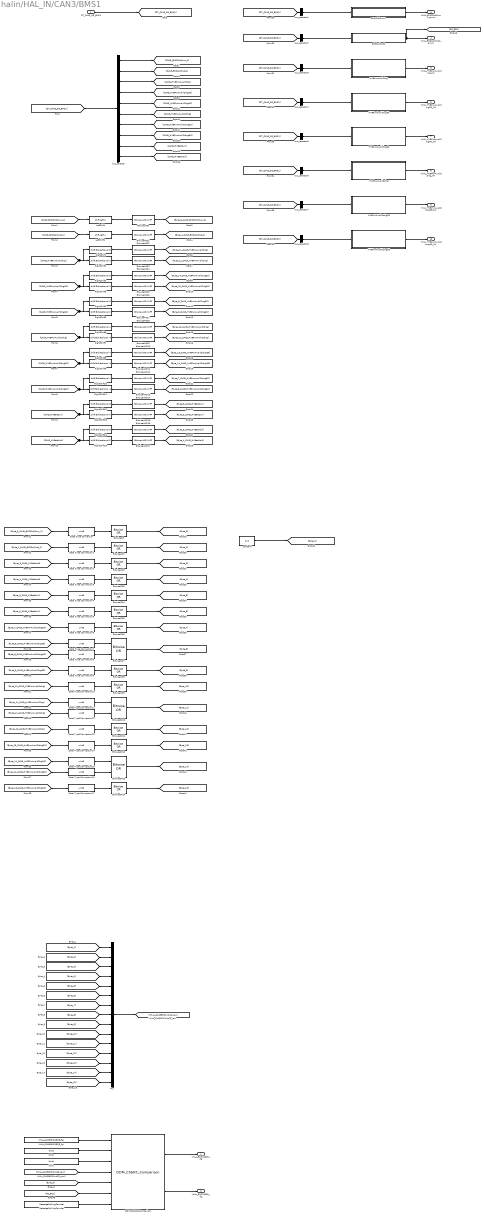
== system halin/HAL_IN/CAN3/BMS1 ==
  DT_CAN3_SG_BMS1 : Inport
  0x3c : Constant  Value=0x3c
  0xdc : Constant  Value=0xdc
  BMSChckSum1 : Subsystem
  BMSRolCnct1 : Subsystem
  BitwiseAND{,1..17} (18 alike) : simulink/Logic and Bit Operations/Bitwise Operator  logicop=AND  UseBitMask=on  BitMask=0xFF  BitMaskRealWorld=Stored Integer
  BitwiseOR{,1..6,8..9,11..12,14} (12 alike) : simulink/Logic and Bit Operations/Bitwise Operator  logicop=OR  UseBitMask=off  BitMask=bin2dec('11011001')  BitMaskRealWorld=Stored Integer
  BitwiseOR10 : simulink/Logic and Bit Operations/Bitwise Operator  logicop=OR  UseBitMask=off  NumInputPorts=2  BitMask=bin2dec('11011001')  BitMaskRealWorld=Stored Integer
  BitwiseOR13 : simulink/Logic and Bit Operations/Bitwise Operator  logicop=OR  UseBitMask=off  NumInputPorts=2  BitMask=bin2dec('11011001')  BitMaskRealWorld=Stored Integer
  BitwiseOR7 : simulink/Logic and Bit Operations/Bitwise Operator  logicop=OR  UseBitMask=off  NumInputPorts=2  BitMask=bin2dec('11011001')  BitMaskRealWorld=Stored Integer
  DDM_CS&RC_Comparison : FVT_lib/hal/DDM_CS&RC_Comparison  MsgCycleTime=10
  Data Type Conversion{,1..17} (18 alike) : DataTypeConversion  OutDataTypeStr=uint8
  HVBPwrAvailChrg : Subsystem
  HVBPwrAvailChrg30 : Subsystem
  HVBPwrAvailChrg60 : Subsystem
  HVBPwrAvailDchrg : Subsystem
  HVBPwrAvailDchrg30 : Subsystem
  HVBPwrAvailDchrg60 : Subsystem
  KHAL_CAN3BMS1E2E_flg : Constant  Value=KHAL_CAN3BMS1E2E_flg
  LeftShift : ArithShift  BitShiftDirection=Left
  LeftShift1 : ArithShift  BitShiftNumber=4  BitShiftDirection=Left
  MessageRollingCounter : FVT_lib/hal/MessageRollingCounter  CounterMAX=14  task_time_ms=5  msg_time_ms=10
  Mux : Mux  Inputs=15
  RightShift{,2,4,12,14} (5 alike) : ArithShift  BitShiftNumber=8
  RightShift{1,3,5,13,15} (5 alike) : ArithShift
  RightShift10 : ArithShift  BitShiftNumber=4
  RightShift11 : ArithShift  BitShiftNumber=-4
  RightShift6 : ArithShift  BitShiftNumber=4
  RightShift7 : ArithShift  BitShiftNumber=-4
  RightShift8 : ArithShift  BitShiftNumber=4
  RightShift9 : ArithShift  BitShiftNumber=-4
  bus_selector : BusSelector  OutputSignals=CAN3_BMSChckSum_1,CAN3_BMSRolCnct_1,CAN3_HVBPwrAvailChrg,CAN3_HVBPwrAvailChrg30,CAN3_HVBPwrAvailChrg60,CAN3_HVBPwrAvailDchrg,CAN3_HVBPwrAvailDchrg30,CAN3_HVBPwrAvailDchrg60,CAN3_HVBattCurr,CAN3_HVBattVolt
  bus_selector1 : BusSelector  OutputSignals=CAN3_BMSChckSum_1
  bus_selector2 : BusSelector  OutputSignals=CAN3_BMSRolCnct_1
  bus_selector3 : BusSelector  OutputSignals=CAN3_HVBPwrAvailChrg
  bus_selector4 : BusSelector  OutputSignals=CAN3_HVBPwrAvailChrg30
  bus_selector5 : BusSelector  OutputSignals=CAN3_HVBPwrAvailChrg60
  bus_selector6 : BusSelector  OutputSignals=CAN3_HVBPwrAvailDchrg
  bus_selector7 : BusSelector  OutputSignals=CAN3_HVBPwrAvailDchrg30
  bus_selector8 : BusSelector  OutputSignals=CAN3_HVBPwrAvailDchrg60
  constant : Constant  Value=0x0  OutDataTypeStr=uint8
  VHAL_BMS1CSErr_flg : Outport
  VHAL_BMS1RCErr_flg : Outport  Port=2
  VHAL_BMSChckSum1_enum : Outport  Port=3
  VHAL_BMSRolCnct1_enum : Outport  Port=4
  VHAL_HVBPwrAvailChrg_kW : Outport  Port=5
  VHAL_HVBPwrAvailChrg30_kW : Outport  Port=6
  VHAL_HVBPwrAvailChrg60_kW : Outport  Port=7
  VHAL_HVBPwrAvailDchrg_kW : Outport  Port=8
  VHAL_HVBPwrAvailDchrg30_kW : Outport  Port=9
  VHAL_HVBPwrAvailDchrg60_kW : Outport  Port=10
  wires:
  DT_CAN3_SG_BMS1/1 -> [DT_CAN3_SG_BMS1]
  [DT_CAN3_SG_BMS1] -> bus_selector/1
  bus_selector/1 -> [CAN3_BMSChckSum_1]  "<CAN3_BMSChckSum_1>"
  [CAN3_BMSChckSum_1] -> LeftShift/1
  LeftShift/1 -> BitwiseAND/1
  BitwiseAND/1 -> [Byte_0_CAN3_BMSChckSum_1]
  bus_selector/2 -> [CAN3_BMSRolCnct_1]  "<CAN3_BMSRolCnct_1>"
  [CAN3_BMSRolCnct_1] -> LeftShift1/1
  LeftShift1/1 -> BitwiseAND1/1
  BitwiseAND1/1 -> [Byte_1_CAN3_BMSRolCnct_1]
  bus_selector/3 -> [CAN3_HVBPwrAvailChrg]  "<CAN3_HVBPwrAvailChrg>"
  [CAN3_HVBPwrAvailChrg] -> RightShift/1, RightShift1/1
  RightShift/1 -> BitwiseAND2/1
  BitwiseAND2/1 -> [Byte_11_CAN3_HVBPwrAvailChrg]
  RightShift1/1 -> BitwiseAND3/1
  BitwiseAND3/1 -> [Byte_12_CAN3_HVBPwrAvailChrg]
  bus_selector/4 -> [CAN3_HVBPwrAvailChrg30]  "<CAN3_HVBPwrAvailChrg30>"
  [CAN3_HVBPwrAvailChrg30] -> RightShift2/1, RightShift3/1
  RightShift2/1 -> BitwiseAND4/1
  BitwiseAND4/1 -> [Byte_14_CAN3_HVBPwrAvailChrg30]
  RightShift3/1 -> BitwiseAND5/1
  BitwiseAND5/1 -> [Byte_15_CAN3_HVBPwrAvailChrg30]
  bus_selector/5 -> [CAN3_HVBPwrAvailChrg60]  "<CAN3_HVBPwrAvailChrg60>"
  [CAN3_HVBPwrAvailChrg60] -> RightShift4/1, RightShift5/1
  RightShift4/1 -> BitwiseAND6/1
  BitwiseAND6/1 -> [Byte_8_CAN3_HVBPwrAvailChrg60]
  RightShift5/1 -> BitwiseAND7/1
  BitwiseAND7/1 -> [Byte_9_CAN3_HVBPwrAvailChrg60]
  bus_selector/6 -> [CAN3_HVBPwrAvailDchrg]  "<CAN3_HVBPwrAvailDchrg>"
  [CAN3_HVBPwrAvailDchrg] -> RightShift6/1, RightShift7/1
  RightShift6/1 -> BitwiseAND8/1
  BitwiseAND8/1 -> [Byte_10_CAN3_HVBPwrAvailDchrg]
  RightShift7/1 -> BitwiseAND9/1
  BitwiseAND9/1 -> [Byte_11_CAN3_HVBPwrAvailDchrg]
  bus_selector/7 -> [CAN3_HVBPwrAvailDchrg30]  "<CAN3_HVBPwrAvailDchrg30>"
  [CAN3_HVBPwrAvailDchrg30] -> RightShift8/1, RightShift9/1
  RightShift8/1 -> BitwiseAND10/1
  BitwiseAND10/1 -> [Byte_13_CAN3_HVBPwrAvailDchrg30]
  RightShift9/1 -> BitwiseAND11/1
  BitwiseAND11/1 -> [Byte_14_CAN3_HVBPwrAvailDchrg30]
  bus_selector/8 -> [CAN3_HVBPwrAvailDchrg60]  "<CAN3_HVBPwrAvailDchrg60>"
  [CAN3_HVBPwrAvailDchrg60] -> RightShift10/1, RightShift11/1
  RightShift10/1 -> BitwiseAND12/1
  BitwiseAND12/1 -> [Byte_7_CAN3_HVBPwrAvailDchrg60]
  RightShift11/1 -> BitwiseAND13/1
  BitwiseAND13/1 -> [Byte_8_CAN3_HVBPwrAvailDchrg60]
  bus_selector/9 -> [CAN3_HVBattCurr]  "<CAN3_HVBattCurr>"
  [CAN3_HVBattCurr] -> RightShift12/1, RightShift13/1
  RightShift12/1 -> BitwiseAND14/1
  BitwiseAND14/1 -> [Byte_5_CAN3_HVBattCurr]
  RightShift13/1 -> BitwiseAND15/1
  BitwiseAND15/1 -> [Byte_6_CAN3_HVBattCurr]
  bus_selector/10 -> [CAN3_HVBattVolt]  "<CAN3_HVBattVolt>"
  [CAN3_HVBattVolt] -> RightShift14/1, RightShift15/1
  RightShift14/1 -> BitwiseAND16/1
  BitwiseAND16/1 -> [Byte_3_CAN3_HVBattVolt]
  RightShift15/1 -> BitwiseAND17/1
  BitwiseAND17/1 -> [Byte_4_CAN3_HVBattVolt]
  Data Type Conversion/1 -> BitwiseOR/1
  [Byte_0_CAN3_BMSChckSum_1] -> Data Type Conversion/1
  BitwiseOR/1 -> [Byte_0]
  Data Type Conversion1/1 -> BitwiseOR1/1
  [Byte_1_CAN3_BMSRolCnct_1] -> Data Type Conversion1/1
  BitwiseOR1/1 -> [Byte_1]
  constant/1 -> [Byte_2]
  Data Type Conversion2/1 -> BitwiseOR2/1
  [Byte_3_CAN3_HVBattVolt] -> Data Type Conversion2/1
  BitwiseOR2/1 -> [Byte_3]
  Data Type Conversion3/1 -> BitwiseOR3/1
  [Byte_4_CAN3_HVBattVolt] -> Data Type Conversion3/1
  BitwiseOR3/1 -> [Byte_4]
  Data Type Conversion4/1 -> BitwiseOR4/1
  [Byte_5_CAN3_HVBattCurr] -> Data Type Conversion4/1
  BitwiseOR4/1 -> [Byte_5]
  Data Type Conversion5/1 -> BitwiseOR5/1
  [Byte_6_CAN3_HVBattCurr] -> Data Type Conversion5/1
  BitwiseOR5/1 -> [Byte_6]
  Data Type Conversion6/1 -> BitwiseOR6/1
  [Byte_7_CAN3_HVBPwrAvailDchrg60] -> Data Type Conversion6/1
  BitwiseOR6/1 -> [Byte_7]
  Data Type Conversion7/1 -> BitwiseOR7/1
  [Byte_8_CAN3_HVBPwrAvailChrg60] -> Data Type Conversion7/1
  Data Type Conversion8/1 -> BitwiseOR7/2
  [Byte_8_CAN3_HVBPwrAvailDchrg60] -> Data Type Conversion8/1
  BitwiseOR7/1 -> [Byte_8]
  Data Type Conversion9/1 -> BitwiseOR8/1
  [Byte_9_CAN3_HVBPwrAvailChrg60] -> Data Type Conversion9/1
  BitwiseOR8/1 -> [Byte_9]
  Data Type Conversion10/1 -> BitwiseOR9/1
  [Byte_10_CAN3_HVBPwrAvailDchrg] -> Data Type Conversion10/1
  BitwiseOR9/1 -> [Byte_10]
  Data Type Conversion11/1 -> BitwiseOR10/1
  [Byte_11_CAN3_HVBPwrAvailChrg] -> Data Type Conversion11/1
  Data Type Conversion12/1 -> BitwiseOR10/2
  [Byte_11_CAN3_HVBPwrAvailDchrg] -> Data Type Conversion12/1
  BitwiseOR10/1 -> [Byte_11]
  Data Type Conversion13/1 -> BitwiseOR11/1
  [Byte_12_CAN3_HVBPwrAvailChrg] -> Data Type Conversion13/1
  BitwiseOR11/1 -> [Byte_12]
  Data Type Conversion14/1 -> BitwiseOR12/1
  [Byte_13_CAN3_HVBPwrAvailDchrg30] -> Data Type Conversion14/1
  BitwiseOR12/1 -> [Byte_13]
  Data Type Conversion15/1 -> BitwiseOR13/1
  [Byte_14_CAN3_HVBPwrAvailChrg30] -> Data Type Conversion15/1
  Data Type Conversion16/1 -> BitwiseOR13/2
  [Byte_14_CAN3_HVBPwrAvailDchrg30] -> Data Type Conversion16/1
  BitwiseOR13/1 -> [Byte_14]
  Data Type Conversion17/1 -> BitwiseOR14/1
  [Byte_15_CAN3_HVBPwrAvailChrg30] -> Data Type Conversion17/1
  BitwiseOR14/1 -> [Byte_15]
  [Byte_1] -> Mux/1
  [Byte_2] -> Mux/2
  [Byte_3] -> Mux/3
  [Byte_4] -> Mux/4
  [Byte_5] -> Mux/5
  [Byte_6] -> Mux/6
  [Byte_7] -> Mux/7
  [Byte_8] -> Mux/8
  [Byte_9] -> Mux/9
  [Byte_10] -> Mux/10
  [Byte_11] -> Mux/11
  [Byte_12] -> Mux/12
  [Byte_13] -> Mux/13
  [Byte_14] -> Mux/14
  [Byte_15] -> Mux/15
  Mux/1 -> [VHAL_CAN3BMS1noCS_raw]
  KHAL_CAN3BMS1E2E_flg/1 -> DDM_CS&RC_Comparison/1
  0x3c/1 -> DDM_CS&RC_Comparison/2
  0xdc/1 -> DDM_CS&RC_Comparison/3
  [VHAL_CAN3BMS1noCS_raw] -> DDM_CS&RC_Comparison/4
  [Byte_0] -> DDM_CS&RC_Comparison/5
  [RC_ECU] -> DDM_CS&RC_Comparison/6
  MessageRollingCounter/1 -> DDM_CS&RC_Comparison/7
  DDM_CS&RC_Comparison/1 -> VHAL_BMS1CSErr_flg/1
  DDM_CS&RC_Comparison/2 -> VHAL_BMS1RCErr_flg/1
  [DT_CAN3_SG_BMS1] -> bus_selector1/1
  bus_selector1/1 -> BMSChckSum1/1(BMSChckSum_1)  "<CAN3_BMSChckSum_1>"
  BMSChckSum1/1(VHAL_BMSChckSum1_enum) -> VHAL_BMSChckSum1_enum/1
  [DT_CAN3_SG_BMS1] -> bus_selector2/1
  bus_selector2/1 -> BMSRolCnct1/1(BMSRolCnct_1)  "<CAN3_BMSRolCnct_1>"
  BMSRolCnct1/1(VHAL_BMSRolCnct1_enum) -> VHAL_BMSRolCnct1_enum/1, [RC_ECU]
  [DT_CAN3_SG_BMS1] -> bus_selector3/1
  bus_selector3/1 -> HVBPwrAvailChrg/1(HVBPwrAvailChrg)  "<CAN3_HVBPwrAvailChrg>"
  HVBPwrAvailChrg/1(VHAL_HVBPwrAvailChrg_kW) -> VHAL_HVBPwrAvailChrg_kW/1
  [DT_CAN3_SG_BMS1] -> bus_selector4/1
  bus_selector4/1 -> HVBPwrAvailChrg30/1(HVBPwrAvailChrg30)  "<CAN3_HVBPwrAvailChrg30>"
  HVBPwrAvailChrg30/1(VHAL_HVBPwrAvailChrg30_kW) -> VHAL_HVBPwrAvailChrg30_kW/1
  [DT_CAN3_SG_BMS1] -> bus_selector5/1
  bus_selector5/1 -> HVBPwrAvailChrg60/1(HVBPwrAvailChrg60)  "<CAN3_HVBPwrAvailChrg60>"
  HVBPwrAvailChrg60/1(VHAL_HVBPwrAvailChrg60_kW) -> VHAL_HVBPwrAvailChrg60_kW/1
  [DT_CAN3_SG_BMS1] -> bus_selector6/1
  bus_selector6/1 -> HVBPwrAvailDchrg/1(HVBPwrAvailDchrg)  "<CAN3_HVBPwrAvailDchrg>"
  HVBPwrAvailDchrg/1(VHAL_HVBPwrAvailDchrg_kW) -> VHAL_HVBPwrAvailDchrg_kW/1
  [DT_CAN3_SG_BMS1] -> bus_selector7/1
  bus_selector7/1 -> HVBPwrAvailDchrg30/1(HVBPwrAvailDchrg30)  "<CAN3_HVBPwrAvailDchrg30>"
  HVBPwrAvailDchrg30/1(VHAL_HVBPwrAvailDchrg30_kW) -> VHAL_HVBPwrAvailDchrg30_kW/1
  [DT_CAN3_SG_BMS1] -> bus_selector8/1
  bus_selector8/1 -> HVBPwrAvailDchrg60/1(HVBPwrAvailDchrg60)  "<CAN3_HVBPwrAvailDchrg60>"
  HVBPwrAvailDchrg60/1(VHAL_HVBPwrAvailDchrg60_kW) -> VHAL_HVBPwrAvailDchrg60_kW/1

== system halin/HAL_IN/CAN3/BMS2 ==
  DT_CAN3_SG_BMS2 : Inport
  HVInVolt : Subsystem
  LVBattDet12V : Subsystem
  OBCDCCurLm : Subsystem
  OBCDCVoltLm : Subsystem
  bus_selector : BusSelector  OutputSignals=CAN3_HVInVolt
  bus_selector1 : BusSelector  OutputSignals=CAN3_LVBattDet12V
  bus_selector2 : BusSelector  OutputSignals=CAN3_OBCDCCurLm
  bus_selector3 : BusSelector  OutputSignals=CAN3_OBCDCVoltLm
  VHAL_HVInVolt_V : Outport
  VHAL_LVBattDet12V_V : Outport  Port=2
  VHAL_OBCDCCurLm_A : Outport  Port=3
  VHAL_OBCDCVoltLm_V : Outport  Port=4
  wires:
  DT_CAN3_SG_BMS2/1 -> [DT_CAN3_SG_BMS2]
  [DT_CAN3_SG_BMS2] -> bus_selector/1
  bus_selector/1 -> HVInVolt/1(HVInVolt)  "<CAN3_HVInVolt>"
  HVInVolt/1(VHAL_HVInVolt_V) -> VHAL_HVInVolt_V/1
  [DT_CAN3_SG_BMS2] -> bus_selector1/1
  bus_selector1/1 -> LVBattDet12V/1(LVBattDet12V)  "<CAN3_LVBattDet12V>"
  LVBattDet12V/1(VHAL_LVBattDet12V_V) -> VHAL_LVBattDet12V_V/1
  [DT_CAN3_SG_BMS2] -> bus_selector2/1
  bus_selector2/1 -> OBCDCCurLm/1(OBCDCCurLm)  "<CAN3_OBCDCCurLm>"
  OBCDCCurLm/1(VHAL_OBCDCCurLm_A) -> VHAL_OBCDCCurLm_A/1
  [DT_CAN3_SG_BMS2] -> bus_selector3/1
  bus_selector3/1 -> OBCDCVoltLm/1(OBCDCVoltLm)  "<CAN3_OBCDCVoltLm>"
  OBCDCVoltLm/1(VHAL_OBCDCVoltLm_V) -> VHAL_OBCDCVoltLm_V/1

== system halin/HAL_IN/CAN3/BMS3 ==
  DT_CAN3_SG_BMS3 : Inport
  ACChrgCurrDis : Subsystem
  HVBChrgPwr : Subsystem
  HVBChrgPwrTotal : Subsystem
  HVBDrvPwr : Subsystem
  HVBDrvPwrTotal : Subsystem
  HVBFullChrgPwr : Subsystem
  HVBIsoImpedenceN : Subsystem
  HVBIsoImpedenceP : Subsystem
  HVBSOH : Subsystem
  HVBattPackVolt : Subsystem
  HVBattSOC : Subsystem
  HVBattSOCDis : Subsystem
  RemainChrgTime : Subsystem
  bus_selector : BusSelector  OutputSignals=CAN3_ACChrgCurrDis
  bus_selector1 : BusSelector  OutputSignals=CAN3_HVBChrgPwr
  bus_selector10 : BusSelector  OutputSignals=CAN3_HVBattSOC
  bus_selector11 : BusSelector  OutputSignals=CAN3_HVBattSOCDis
  bus_selector12 : BusSelector  OutputSignals=CAN3_RemainChrgTime
  bus_selector2 : BusSelector  OutputSignals=CAN3_HVBChrgPwrTotal
  bus_selector3 : BusSelector  OutputSignals=CAN3_HVBDrvPwr
  bus_selector4 : BusSelector  OutputSignals=CAN3_HVBDrvPwrTotal
  bus_selector5 : BusSelector  OutputSignals=CAN3_HVBFullChrgPwr
  bus_selector6 : BusSelector  OutputSignals=CAN3_HVBIsoImpedenceN
  bus_selector7 : BusSelector  OutputSignals=CAN3_HVBIsoImpedenceP
  bus_selector8 : BusSelector  OutputSignals=CAN3_HVBSOH
  bus_selector9 : BusSelector  OutputSignals=CAN3_HVBattPackVolt
  VHAL_ACChrgCurrDis_A : Outport
  VHAL_HVBChrgPwr_kWh : Outport  Port=2
  VHAL_HVBChrgPwrTotal_kWh : Outport  Port=3
  VHAL_HVBDrvPwr_kWh : Outport  Port=4
  VHAL_HVBDrvPwrTotal_kWh : Outport  Port=5
  VHAL_HVBFullChrgPwr_kWh : Outport  Port=6
  VHAL_HVBIsoImpedenceN_Megaohm : Outport  Port=7
  VHAL_HVBIsoImpedenceP_Megaohm : Outport  Port=8
  VHAL_HVBSOH_pct : Outport  Port=9
  VHAL_HVBattPackVolt_V : Outport  Port=10
  VHAL_HVBattSOC_pct : Outport  Port=11
  VHAL_HVBattSOCDis_pct : Outport  Port=12
  VHAL_RemainChrgTime_min : Outport  Port=13
  wires:
  DT_CAN3_SG_BMS3/1 -> [DT_CAN3_SG_BMS3]
  [DT_CAN3_SG_BMS3] -> bus_selector/1
  bus_selector/1 -> ACChrgCurrDis/1(ACChrgCurrDis)  "<CAN3_ACChrgCurrDis>"
  ACChrgCurrDis/1(VHAL_ACChrgCurrDis_A) -> VHAL_ACChrgCurrDis_A/1
  [DT_CAN3_SG_BMS3] -> bus_selector1/1
  bus_selector1/1 -> HVBChrgPwr/1(HVBChrgPwr)  "<CAN3_HVBChrgPwr>"
  HVBChrgPwr/1(VHAL_HVBChrgPwr_kWh) -> VHAL_HVBChrgPwr_kWh/1
  [DT_CAN3_SG_BMS3] -> bus_selector2/1
  bus_selector2/1 -> HVBChrgPwrTotal/1(HVBChrgPwrTotal)  "<CAN3_HVBChrgPwrTotal>"
  HVBChrgPwrTotal/1(VHAL_HVBChrgPwrTotal_kWh) -> VHAL_HVBChrgPwrTotal_kWh/1
  [DT_CAN3_SG_BMS3] -> bus_selector3/1
  bus_selector3/1 -> HVBDrvPwr/1(HVBDrvPwr)  "<CAN3_HVBDrvPwr>"
  HVBDrvPwr/1(VHAL_HVBDrvPwr_kWh) -> VHAL_HVBDrvPwr_kWh/1
  [DT_CAN3_SG_BMS3] -> bus_selector4/1
  bus_selector4/1 -> HVBDrvPwrTotal/1(HVBDrvPwrTotal)  "<CAN3_HVBDrvPwrTotal>"
  HVBDrvPwrTotal/1(VHAL_HVBDrvPwrTotal_kWh) -> VHAL_HVBDrvPwrTotal_kWh/1
  [DT_CAN3_SG_BMS3] -> bus_selector5/1
  bus_selector5/1 -> HVBFullChrgPwr/1(HVBFullChrgPwr)  "<CAN3_HVBFullChrgPwr>"
  HVBFullChrgPwr/1(VHAL_HVBFullChrgPwr_kWh) -> VHAL_HVBFullChrgPwr_kWh/1
  [DT_CAN3_SG_BMS3] -> bus_selector6/1
  bus_selector6/1 -> HVBIsoImpedenceN/1(HVBIsoImpedenceN)  "<CAN3_HVBIsoImpedenceN>"
  HVBIsoImpedenceN/1(VHAL_HVBIsoImpedenceN_Megaohm) -> VHAL_HVBIsoImpedenceN_Megaohm/1
  [DT_CAN3_SG_BMS3] -> bus_selector7/1
  bus_selector7/1 -> HVBIsoImpedenceP/1(HVBIsoImpedenceP)  "<CAN3_HVBIsoImpedenceP>"
  HVBIsoImpedenceP/1(VHAL_HVBIsoImpedenceP_Megaohm) -> VHAL_HVBIsoImpedenceP_Megaohm/1
  [DT_CAN3_SG_BMS3] -> bus_selector8/1
  bus_selector8/1 -> HVBSOH/1(HVBSOH)  "<CAN3_HVBSOH>"
  HVBSOH/1(VHAL_HVBSOH_pct) -> VHAL_HVBSOH_pct/1
  [DT_CAN3_SG_BMS3] -> bus_selector9/1
  bus_selector9/1 -> HVBattPackVolt/1(HVBattPackVolt)  "<CAN3_HVBattPackVolt>"
  HVBattPackVolt/1(VHAL_HVBattPackVolt_V) -> VHAL_HVBattPackVolt_V/1
  [DT_CAN3_SG_BMS3] -> bus_selector10/1
  bus_selector10/1 -> HVBattSOC/1(HVBattSOC)  "<CAN3_HVBattSOC>"
  HVBattSOC/1(VHAL_HVBattSOC_pct) -> VHAL_HVBattSOC_pct/1
  [DT_CAN3_SG_BMS3] -> bus_selector11/1
  bus_selector11/1 -> HVBattSOCDis/1(HVBattSOCDis)  "<CAN3_HVBattSOCDis>"
  HVBattSOCDis/1(VHAL_HVBattSOCDis_pct) -> VHAL_HVBattSOCDis_pct/1
  [DT_CAN3_SG_BMS3] -> bus_selector12/1
  bus_selector12/1 -> RemainChrgTime/1(RemainChrgTime)  "<CAN3_RemainChrgTime>"
  RemainChrgTime/1(VHAL_RemainChrgTime_min) -> VHAL_RemainChrgTime_min/1

== system halin/HAL_IN/CAN3/BMS4 ==
  DT_CAN3_SG_BMS4 : Inport
  CellTempAvg : Subsystem
  HVBCellVoltMax : Subsystem
  HVBCellVoltMin : Subsystem
  HVBMTempMax : Subsystem
  HVBMTempMin : Subsystem
  MaxCellTempNum : Subsystem
  MaxCellVoltNum : Subsystem
  MinCellTempNum : Subsystem
  MinCellVoltNum : Subsystem
  bus_selector : BusSelector  OutputSignals=CAN3_CellTempAvg
  bus_selector1 : BusSelector  OutputSignals=CAN3_HVBCellVoltMax
  bus_selector2 : BusSelector  OutputSignals=CAN3_HVBCellVoltMin
  bus_selector3 : BusSelector  OutputSignals=CAN3_HVBMTempMax
  bus_selector4 : BusSelector  OutputSignals=CAN3_HVBMTempMin
  bus_selector5 : BusSelector  OutputSignals=CAN3_MaxCellTemp_Num
  bus_selector6 : BusSelector  OutputSignals=CAN3_MaxCellVolt_Num
  bus_selector7 : BusSelector  OutputSignals=CAN3_MinCellTemp_Num
  bus_selector8 : BusSelector  OutputSignals=CAN3_MinCellVolt_Num
  VHAL_CellTempAvg_C : Outport
  VHAL_HVBCellVoltMax_mV : Outport  Port=2
  VHAL_HVBCellVoltMin_mV : Outport  Port=3
  VHAL_HVBMTempMax_C : Outport  Port=4
  VHAL_HVBMTempMin_C : Outport  Port=5
  VHAL_MaxCellTempNum_enum : Outport  Port=6
  VHAL_MaxCellVoltNum_enum : Outport  Port=7
  VHAL_MinCellTempNum_enum : Outport  Port=8
  VHAL_MinCellVoltNum_enum : Outport  Port=9
  wires:
  DT_CAN3_SG_BMS4/1 -> [DT_CAN3_SG_BMS4]
  [DT_CAN3_SG_BMS4] -> bus_selector/1
  bus_selector/1 -> CellTempAvg/1(CellTempAvg)  "<CAN3_CellTempAvg>"
  CellTempAvg/1(VHAL_CellTempAvg_C) -> VHAL_CellTempAvg_C/1
  [DT_CAN3_SG_BMS4] -> bus_selector1/1
  bus_selector1/1 -> HVBCellVoltMax/1(HVBCellVoltMax)  "<CAN3_HVBCellVoltMax>"
  HVBCellVoltMax/1(VHAL_HVBCellVoltMax_mV) -> VHAL_HVBCellVoltMax_mV/1
  [DT_CAN3_SG_BMS4] -> bus_selector2/1
  bus_selector2/1 -> HVBCellVoltMin/1(HVBCellVoltMin)  "<CAN3_HVBCellVoltMin>"
  HVBCellVoltMin/1(VHAL_HVBCellVoltMin_mV) -> VHAL_HVBCellVoltMin_mV/1
  [DT_CAN3_SG_BMS4] -> bus_selector3/1
  bus_selector3/1 -> HVBMTempMax/1(HVBMTempMax)  "<CAN3_HVBMTempMax>"
  HVBMTempMax/1(VHAL_HVBMTempMax_C) -> VHAL_HVBMTempMax_C/1
  [DT_CAN3_SG_BMS4] -> bus_selector4/1
  bus_selector4/1 -> HVBMTempMin/1(HVBMTempMin)  "<CAN3_HVBMTempMin>"
  HVBMTempMin/1(VHAL_HVBMTempMin_C) -> VHAL_HVBMTempMin_C/1
  [DT_CAN3_SG_BMS4] -> bus_selector5/1
  bus_selector5/1 -> MaxCellTempNum/1(MaxCellTemp_Num)  "<CAN3_MaxCellTemp_Num>"
  MaxCellTempNum/1(VHAL_MaxCellTempNum_enum) -> VHAL_MaxCellTempNum_enum/1
  [DT_CAN3_SG_BMS4] -> bus_selector6/1
  bus_selector6/1 -> MaxCellVoltNum/1(MaxCellVolt_Num)  "<CAN3_MaxCellVolt_Num>"
  MaxCellVoltNum/1(VHAL_MaxCellVoltNum_enum) -> VHAL_MaxCellVoltNum_enum/1
  [DT_CAN3_SG_BMS4] -> bus_selector7/1
  bus_selector7/1 -> MinCellTempNum/1(MinCellTemp_Num)  "<CAN3_MinCellTemp_Num>"
  MinCellTempNum/1(VHAL_MinCellTempNum_enum) -> VHAL_MinCellTempNum_enum/1
  [DT_CAN3_SG_BMS4] -> bus_selector8/1
  bus_selector8/1 -> MinCellVoltNum/1(MinCellVolt_Num)  "<CAN3_MinCellVolt_Num>"
  MinCellVoltNum/1(VHAL_MinCellVoltNum_enum) -> VHAL_MinCellVoltNum_enum/1
